simulink model "MMP_simulink_prediction_general_example"  (R2019b)
settings: Solver=VariableStepAuto  StartTime=0.0  StopTime=t_run  RelTol=1e-3
values from neighbouring files (symbols this model uses):
  L = 4    [FIR_MMP_example.m]    (also in IIR_MMP_example.m; MMP_prediction_general.m = 6; MMP_simulink.m; MMPexample.m)
  n_amp = 0.001    [MMP_prediction_general.m]    (also in MMP_simulink.m = 0.1; prediction_test.m = 0.03)
  predic_step = 7    [MMP_prediction_general.m]    (also in prediction_test.m = 15)
  Tsf = 0.1    [FIR_MMP_example.m]    (also in IIR_MMP_example.m; MMP_prediction_general.m = 0.008; MMP_simulink.m = 0.025; prediction_test.m = 0.008)
  Tss = Tsf*L    (= 0.4)    [FIR_MMP_example.m]    (also in IIR_MMP_example.m; MMP_prediction_general.m = 0.048; MMP_simulink.m = 0.1; prediction_test.m = 0.048)
  W = FIR_MMP(Apara, L, p)    [FIR_MMP_example.m]    (also in MMP.m = zeros(L-1,m); MMP_prediction_general.m = FIR_MMP(Apara, L, p, predic_step); MMP_simulink.m; MMPexample.m = MMP(Apara, L, p))
libraries: simulink x1
settings Model: Creator=macs  LastModifiedBy=huixiao
settings DataIOCC: ReturnWorkspaceOutputs=off
settings DebuggingCC: ArithmeticOperatorsInVariantConditions=warning
settings SFSimCC: CustomCodeUndefinedFunction=UseInterfaceOnly

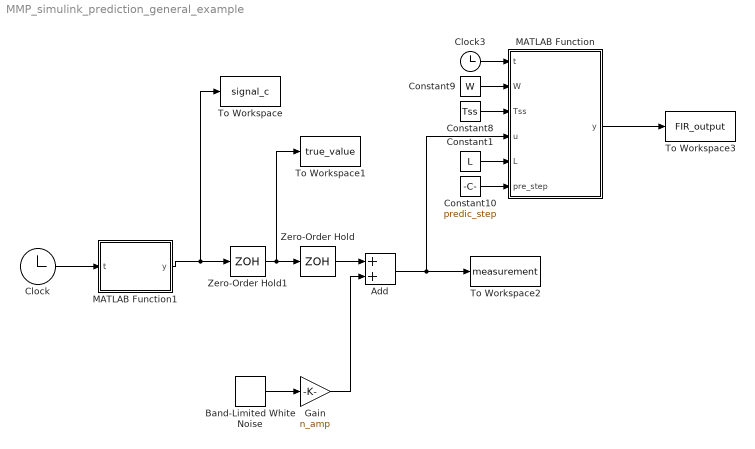
== system MMP_simulink_prediction_general_example ==
  Add : Sum
  Band-Limited White Noise : simulink/Sources/Band-Limited White Noise  Cov=[0.1]  Ts=Tss  seed=[23341]
  Clock : Clock
  Clock3 : Clock
  Constant1 : Constant  Value=L
  Constant10 : Constant  Value=predic_step
  Constant8 : Constant  Value=Tss
  Constant9 : Constant  Value=W
  Gain : Gain  Gain=n_amp
  MATLAB Function : MATLAB Function  TreatAsAtomicUnit=on
  MATLAB Function1 : MATLAB Function  TreatAsAtomicUnit=on
  To Workspace : ToWorkspace  VariableName=signal_c  SaveFormat=Structure With Time  SampleTime=-1
  To Workspace1 : ToWorkspace  VariableName=true_value  SaveFormat=Structure With Time  SampleTime=-1
  To Workspace2 : ToWorkspace  VariableName=measurement  SaveFormat=Structure With Time  SampleTime=-1
  To Workspace3 : ToWorkspace  VariableName=FIR_output  SaveFormat=Structure With Time  SampleTime=-1
  Zero-Order Hold : ZeroOrderHold  SampleTime=Tss
  Zero-Order Hold1 : ZeroOrderHold  SampleTime=Tsf
  wires:
  Band-Limited White Noise/1 -> Gain/1
  MATLAB Function1/1(y) -> To Workspace/1, Zero-Order Hold1/1
  Zero-Order Hold/1 -> Add/1
  Add/1 -> To Workspace2/1, MATLAB Function/4(u)
  Constant1/1 -> MATLAB Function/5(L)
  Constant8/1 -> MATLAB Function/3(Tss)
  Clock3/1 -> MATLAB Function/1(t)
  Constant9/1 -> MATLAB Function/2(W)
  Zero-Order Hold1/1 -> To Workspace1/1, Zero-Order Hold/1
  Gain/1 -> Add/2
  Constant10/1 -> MATLAB Function/6(pre_step)
  Clock/1 -> MATLAB Function1/1(t)
  MATLAB Function/1(y) -> To Workspace3/1

== matlab function MMP_simulink_prediction_general_example/MATLAB Function1 ==
  data: t input; y output
function y = fcn(t)

y = 5*t^2;

== matlab function MMP_simulink_prediction_general_example/MATLAB Function ==
  settings: updateMethod=DISCRETE  sampleTime=Tsf
  data: t input; W input; Tss input; u input; y output; L input; pre_step input
function y = FIR_predictor(t, W, Tss, u, L, pre_step)
% Hui Xiao 10-14-2016
persistent phi;
persistent ulast;
persistent tlast;
[~,m] = size(W);
if isempty(phi)
    phi = zeros(m,1);
    tlast = t;
    ulast = 0;
end

% check if has new input
if(u ~= ulast)
    %update phi
    for i=m:-1:2
        phi(i)=phi(i-1);
    end
    phi(1)=u;
    %update t_last and u_last
    tlast = t;
    ulast = u;
end

% calculate index
Tsf = Tss/L;
idx = round((t-tlast)/Tsf);

% do prediction

y = 0;
for i = 1:m
    if(idx+pre_step == 0)
        % this happens when pre_step=0
        y = u;
    else
        y=y+W(idx+pre_step,i)*phi(i);
        %disp(index)
    end
end

end
